simulink library "nxt_Lib"  (Simulink 7.4)
settings: Solver=ode45  SolverMode=SingleTasking  StartTime=0.0  StopTime=10.0  RelTol=1e-3
libraries: ecrobot_nxt_lib x1, nxt_Lib x1
settings Model: Creator=agerar02  LastModifiedBy=tyler

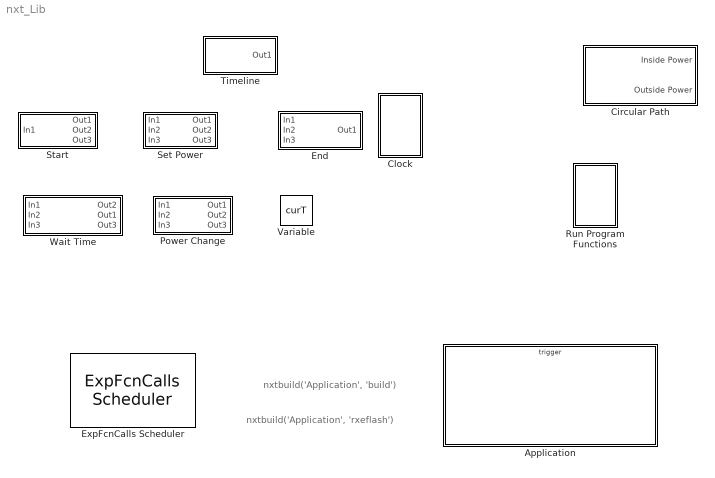
== system nxt_Lib ==
  note: nxtbuild('Application', 'build')
  note: nxtbuild('Application', 'rxeflash')
  Application : Subsystem
  Circular Path : Subsystem  mask(Circular Path  ){a=1, b=.125, c=.08, d=20}
      mask prompts: a "Path Radius"; b "Wheel Base"; c "Wheel Diameter"; d "Speed"
      mask help: Inputs the power to both motors that will cause the ECRobot to run in a Circular Path.
      mask Display: disp('Circular Path')
  Clock : Subsystem  AncestorBlock=nxt_Lib/Timeline/Subsystem6
      mask Type: Clock
      mask Description: Contains the counter
      mask Display: disp('Clock')
  End : Subsystem
      mask Type: End Program
      mask Description: This terminates the time line and passes the final motor speed to the motor. However, it leaves everything running at it's previous power.
      mask Display: disp('End')
  ExpFcnCalls Scheduler : ecrobot_nxt_lib/ExpFcnCalls Scheduler  fcname='fcn'  fctrigger=[1]  ts=0.001  platform=OSEK  stacksize=[512]  bd_mode=Slave
  Power Change : Subsystem  mask(Power Change){c=60}
      mask prompts: c "Power Change"
      mask help: This will add or subtract from the power amount
      mask Display: disp('Power Change')
  Run Program Functions : Subsystem
  Set Power : Subsystem  mask(Set Power){a=60}
      mask prompts: a "Set Power"
      mask help: This box sets the power
      mask Display: disp('Set Power')
  Start : Subsystem
      mask Type: Start
      mask Description: Initializes the timeline
      mask Display: disp('Start')
  Timeline : Subsystem  AncestorBlock=nxt_Lib/Timeline
  Variable : DataStoreMemory  DataStoreName=curT  ReadBeforeWriteMsg=warning  WriteAfterWriteMsg=warning  WriteAfterReadMsg=warning  OutDataType=fixdt(1, 16)  OutScaling=2^0
  Wait Time : Subsystem  mask(Wait Time){b=3}
      mask prompts: b "Wait Time (seconds)"
      mask Display: disp('Wait Time')

== system nxt_Lib/Application ==
  function : TriggerPort  TriggerType=function-call
  Data Store Memory : DataStoreMemory  DataStoreName=curT  ReadBeforeWriteMsg=warning  WriteAfterWriteMsg=warning  WriteAfterReadMsg=warning  OutDataType=fixdt(1, 16)  OutScaling=2^0
  Subsystem6 : Subsystem  AncestorBlock=nxt_Lib/Timeline/Subsystem6
      mask Type: Clock
      mask Description: Contains the counter
      mask Display: disp('Clock')

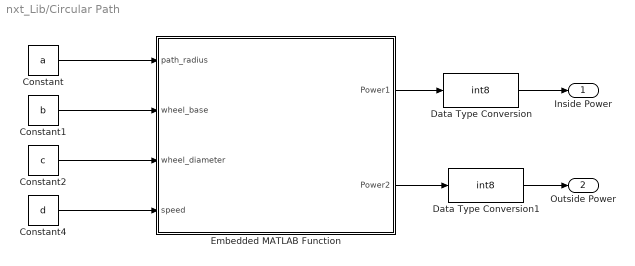
== system nxt_Lib/Circular Path ==
  Constant : Constant  Value=a  OutDataTypeMode=single  OutDataType=sfix(16)  OutScaling=2^0  OutDataTypeStr=single  SampleTime=-1
  Constant1 : Constant  Value=b  OutDataTypeMode=single  OutDataType=sfix(16)  OutScaling=2^0  OutDataTypeStr=single  SampleTime=-1
  Constant2 : Constant  Value=c  OutDataTypeMode=single  OutDataType=sfix(16)  OutScaling=2^0  OutDataTypeStr=single  SampleTime=-1
  Constant4 : Constant  Value=d  OutDataTypeMode=single  OutDataType=sfix(16)  OutScaling=2^0  OutDataTypeStr=single  SampleTime=-1
  Data Type Conversion : DataTypeConversion  OutDataTypeMode=int8  OutDataType=sfix(16)  OutScaling=2^0  OutDataTypeStr=int8
  Data Type Conversion1 : DataTypeConversion  OutDataTypeMode=int8  OutDataType=sfix(16)  OutScaling=2^0  OutDataTypeStr=int8
  Embedded MATLAB Function : Stateflow chart
  Inside Power : Outport
  Outside Power : Outport  Port=2
  wires:
  Embedded MATLAB Function/2(Power2) -> Data Type Conversion1/1
  Embedded MATLAB Function/1(Power1) -> Data Type Conversion/1
  Constant4/1 -> Embedded MATLAB Function/4(speed)
  Constant2/1 -> Embedded MATLAB Function/3(wheel_diameter)
  Constant1/1 -> Embedded MATLAB Function/2(wheel_base)
  Constant/1 -> Embedded MATLAB Function/1(path_radius)
  Data Type Conversion/1 -> Inside Power/1
  Data Type Conversion1/1 -> Outside Power/1

== system nxt_Lib/Clock ==
  Data Store Write : DataStoreWrite  DataStoreName=curT  SampleTime=-1
  Subsystem : Subsystem
      mask Type: Clock
      mask Description: Increments a counter that acts as a clock that changes per unit time.
      mask Display: disp('Clock')
  wires:
  Subsystem/1(Out1) -> Data Store Write/1

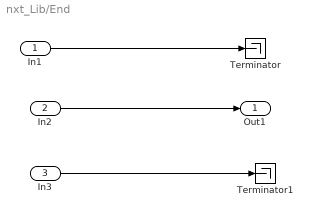
== system nxt_Lib/End ==
  In1 : Inport
  In2 : Inport  Port=2  DataType=int32  OutDataTypeStr=int32
  In3 : Inport  Port=3
  Terminator : Terminator
  Terminator1 : Terminator
  Out1 : Outport
  wires:
  In3/1 -> Terminator1/1
  In1/1 -> Terminator/1
  In2/1 -> Out1/1

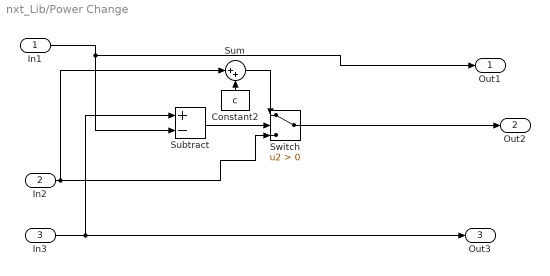
== system nxt_Lib/Power Change ==
  In1 : Inport
  In2 : Inport  Port=2
  In3 : Inport  Port=3
  Constant2 : Constant  Value=c  OutDataTypeMode=int32  OutDataType=fixdt(1, 16)  OutScaling=2^0  OutDataTypeStr=int32  SampleTime=-1
  Subtract : Sum  Inputs=+-  OutDataType=fixdt(1, 16)  OutScaling=2^-10
  Sum : Sum  Inputs=|++  OutDataType=sfix(16)  OutScaling=2^0
  Switch : Switch  Criteria=u2 > Threshold  OutDataType=fixdt(1, 16)  OutScaling=2^0
  Out1 : Outport
  Out2 : Outport  Port=2
  Out3 : Outport  Port=3
  wires:
  Constant2/1 -> Sum/2
  In2/1 -> Sum/1, Switch/3
  Sum/1 -> Switch/1
  Switch/1 -> Out2/1
  Subtract/1 -> Switch/2
  In3/1 -> Out3/1, Subtract/1
  In1/1 -> Out1/1, Subtract/2

== system nxt_Lib/Run Program Functions ==
  note: nxtconfig(gcs)
  note: nxtbuild('Motor3_app', 'rxeflash')
  note: nxtbuild('Motor3_app', 'build')
  note: Drag these blocks to the main model page.

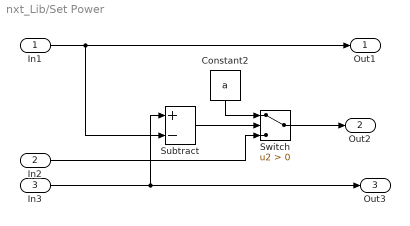
== system nxt_Lib/Set Power ==
  In1 : Inport
  In2 : Inport  Port=2
  In3 : Inport  Port=3
  Constant2 : Constant  Value=a  OutDataTypeMode=int32  OutDataType=fixdt(1, 16)  OutScaling=2^0  OutDataTypeStr=int32  SampleTime=-1
  Subtract : Sum  Inputs=+-  OutDataType=fixdt(1, 16)  OutScaling=2^-10  OutDataTypeStr=Inherit: Same as first input
  Switch : Switch  Criteria=u2 > Threshold  OutDataType=fixdt(1, 16)  OutScaling=2^0
  Out1 : Outport
  Out2 : Outport  Port=2
  Out3 : Outport  Port=3
  wires:
  In2/1 -> Switch/3
  Constant2/1 -> Switch/1
  Switch/1 -> Out2/1
  Subtract/1 -> Switch/2
  In3/1 -> Out3/1, Subtract/1
  In1/1 -> Out1/1, Subtract/2

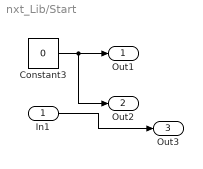
== system nxt_Lib/Start ==
  In1 : Inport
  Constant3 : Constant  Value=0  OutDataTypeMode=int32  OutDataType=fixdt(1, 16)  OutScaling=2^0  OutDataTypeStr=int32  SampleTime=1
  Out1 : Outport
  Out2 : Outport  Port=2
  Out3 : Outport  Port=3
  wires:
  In1/1 -> Out3/1
  Constant3/1 -> Out2/1, Out1/1

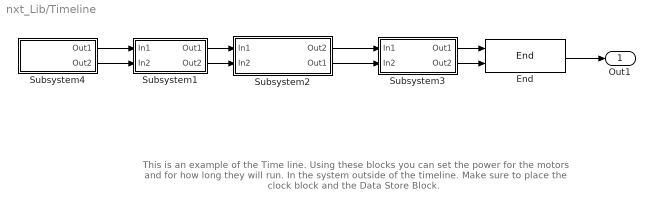
== system nxt_Lib/Timeline ==
  note: This is an example of the Time line. Using these blocks you can set the power for the motors
      | and for how long they will run. In the system outside of the timeline. Make sure to place the clock block and the Data Store Block.
  End : nxt_Lib/End  SystemSampleTime=-1
  Subsystem1 : Subsystem  mask(Set Power){a=0}
      mask prompts: a "Set Power"
      mask help: This box sets the power
      mask Display: disp('Set Power')
  Subsystem2 : Subsystem  mask(Wait Time){b=5000}
      mask prompts: b "Wait Time (seconds)"
      mask Display: disp('Wait Time')
  Subsystem3 : Subsystem  mask(Power Change){c=100}
      mask prompts: c "Power Change"
      mask help: This will add or subtract from the power amount
      mask Display: disp('Power Change')
  Subsystem4 : Subsystem
      mask Type: Start
      mask Description: Initializes the timeline
      mask Display: disp('Start')
  Out1 : Outport
  wires:
  Subsystem3/2(Out2) -> End/2
  Subsystem3/1(Out1) -> End/1
  Subsystem4/2(Out2) -> Subsystem1/2(In2)
  Subsystem4/1(Out1) -> Subsystem1/1(In1)
  Subsystem1/2(Out2) -> Subsystem2/2(In2)
  Subsystem1/1(Out1) -> Subsystem2/1(In1)
  Subsystem2/2(Out1) -> Subsystem3/2(In2)
  Subsystem2/1(Out2) -> Subsystem3/1(In1)
  End/1 -> Out1/1

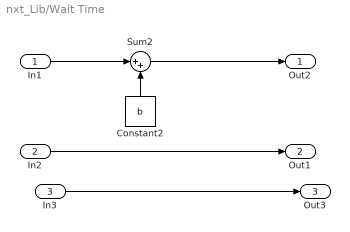
== system nxt_Lib/Wait Time ==
  In1 : Inport
  In2 : Inport  Port=2
  In3 : Inport  Port=3
  Constant2 : Constant  Value=b  OutDataTypeMode=int32  OutDataType=fixdt(1, 16)  OutScaling=2^0  OutDataTypeStr=int32  SampleTime=-1
  Sum2 : Sum  Inputs=|++  OutDataType=fixdt(1, 16)  OutScaling=2^0  OutDataTypeStr=Inherit: Same as first input
  Out2 : Outport
  Out1 : Outport  Port=2
  Out3 : Outport  Port=3
  wires:
  In3/1 -> Out3/1
  In2/1 -> Out1/1
  Sum2/1 -> Out2/1
  Constant2/1 -> Sum2/2
  In1/1 -> Sum2/1

== system nxt_Lib/Application/Subsystem6 ==
  Data Store Write : DataStoreWrite  DataStoreName=curT  SampleTime=-1
  Subsystem : Subsystem
      mask Type: Clock
      mask Description: Increments a counter that acts as a clock that changes per unit time.
      mask Display: disp('Clock')
  wires:
  Subsystem/1(Out1) -> Data Store Write/1

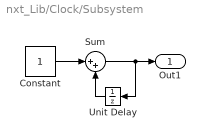
== system nxt_Lib/Clock/Subsystem ==
  Constant : Constant  OutDataTypeMode=int32  OutDataType=fixdt(1, 16)  OutScaling=2^0  OutDataTypeStr=int32  SampleTime=-1
  Sum : Sum  Inputs=|++  AccumDataTypeStr=int8  OutDataType=fixdt(1, 16)  OutScaling=2^0  OutDataTypeStr=Inherit: Same as first input
  Unit Delay : UnitDelay  SampleTime=-1
  Out1 : Outport
  wires:
  Constant/1 -> Sum/1
  Sum/1 -> Unit Delay/1, Out1/1
  Unit Delay/1 -> Sum/2

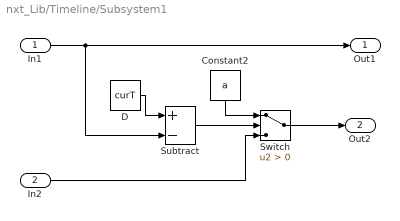
== system nxt_Lib/Timeline/Subsystem1 ==
  In1 : Inport
  In2 : Inport  Port=2
  Constant2 : Constant  Value=a  OutDataTypeMode=int8  OutDataType=fixdt(1, 16)  OutScaling=2^0  OutDataTypeStr=int8  SampleTime=-1
  D : DataStoreRead  DataStoreName=curT  SampleTime=-1
  Subtract : Sum  Inputs=+-  OutDataType=fixdt(1, 16)  OutScaling=2^-10  OutDataTypeStr=Inherit: Same as first input
  Switch : Switch  Criteria=u2 > Threshold  OutDataType=fixdt(1, 16)  OutScaling=2^0
  Out1 : Outport
  Out2 : Outport  Port=2
  wires:
  In2/1 -> Switch/3
  Constant2/1 -> Switch/1
  Switch/1 -> Out2/1
  Subtract/1 -> Switch/2
  D/1 -> Subtract/1
  In1/1 -> Out1/1, Subtract/2

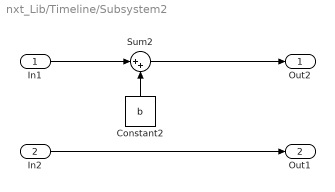
== system nxt_Lib/Timeline/Subsystem2 ==
  In1 : Inport
  In2 : Inport  Port=2
  Constant2 : Constant  Value=b  OutDataTypeMode=int32  OutDataType=fixdt(1, 16)  OutScaling=2^0  OutDataTypeStr=int32  SampleTime=-1
  Sum2 : Sum  Inputs=|++  OutDataType=fixdt(1, 16)  OutScaling=2^0  OutDataTypeStr=Inherit: Same as first input
  Out2 : Outport
  Out1 : Outport  Port=2
  wires:
  In2/1 -> Out1/1
  Sum2/1 -> Out2/1
  Constant2/1 -> Sum2/2
  In1/1 -> Sum2/1

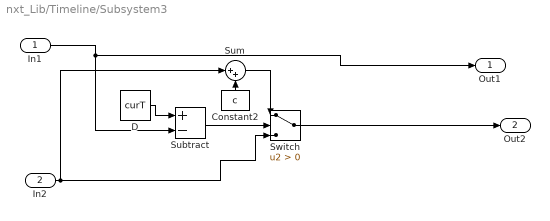
== system nxt_Lib/Timeline/Subsystem3 ==
  In1 : Inport
  In2 : Inport  Port=2
  Constant2 : Constant  Value=c  OutDataTypeMode=int32  OutDataType=fixdt(1, 16)  OutScaling=2^0  OutDataTypeStr=int32  SampleTime=-1
  D : DataStoreRead  DataStoreName=curT  SampleTime=-1
  Subtract : Sum  Inputs=+-  OutDataType=fixdt(1, 16)  OutScaling=2^-10
  Sum : Sum  Inputs=|++  OutDataType=sfix(16)  OutScaling=2^0
  Switch : Switch  Criteria=u2 > Threshold  OutDataType=fixdt(1, 16)  OutScaling=2^0
  Out1 : Outport
  Out2 : Outport  Port=2
  wires:
  Constant2/1 -> Sum/2
  In2/1 -> Sum/1, Switch/3
  Sum/1 -> Switch/1
  Switch/1 -> Out2/1
  Subtract/1 -> Switch/2
  D/1 -> Subtract/1
  In1/1 -> Out1/1, Subtract/2

== system nxt_Lib/Timeline/Subsystem4 ==
  Constant3 : Constant  Value=0  OutDataTypeMode=int32  OutDataType=fixdt(1, 16)  OutScaling=2^0  OutDataTypeStr=int32  SampleTime=-1
  Out1 : Outport
  Out2 : Outport  Port=2
  wires:
  Constant3/1 -> Out2/1, Out1/1

== system nxt_Lib/Application/Subsystem6/Subsystem ==
  Constant : Constant  OutDataTypeMode=int32  OutDataType=fixdt(1, 16)  OutScaling=2^0  OutDataTypeStr=int32  SampleTime=-1
  Sum : Sum  Inputs=|++  AccumDataTypeStr=int8  OutDataType=fixdt(1, 16)  OutScaling=2^0  OutDataTypeStr=Inherit: Same as first input
  Unit Delay : UnitDelay  SampleTime=-1
  Out1 : Outport
  wires:
  Unit Delay/1 -> Sum/2
  Sum/1 -> Out1/1, Unit Delay/1
  Constant/1 -> Sum/1

== matlab function Circular Path/Embedded MATLAB Function ==
  data: path_radius input double; Power1 output double; wheel_base input double; wheel_diameter input double; speed input double; Power2 output double
function [Power1, Power2] = circle_path(path_radius,wheel_base,wheel_diameter,speed)
% This block supports the Embedded MATLAB subset.
% See the help menu for details. 

%Wheel one is the inside wheel
%Wheel two is the outside wheel

dis=wheel_base/2;
wheel1_path=path_radius-dis;
wheel2_path=path_radius+dis;

%Calculate the RPM of the car

angular_velocity=speed/path_radius; %This is the angular velocity in radians/min

rpm=angular_velocity/(2*pi); %This is the rpm of the car

%Calculate the linear speed of each wheel

%Inside Wheel
wheel1_speed=rpm*wheel1_path;

%Outside Wheel
wheel2_speed=rpm*wheel2_path;

%Using the linear speeds calculate the rpm of each wheel.

wheel_radius=wheel_diameter/2;

%Inside Wheel
ang_vel1=wheel1_speed/wheel_radius;
rpm1=ang_vel1/(2*pi);

%Outside Wheel
ang_vel2=wheel2_speed/wheel_radius;
rpm2=ang_vel2/(2*pi);

%Using these rpms and the trendline equation relating rpm to power, get the required power 
%of the wheels.

Power1=.6958*rpm1+1.35709;
Power2=.6958*rpm2+1.35709;
end
